simulink model "SSBWeaverModulatorandDemodulator"  (R2021a)
settings: Solver=VariableStepAuto  StartTime=0.0  StopTime=1  RelTol=1e-3
libraries: dspfdesign x4
settings Model: Creator=ZephyrY  LastModifiedBy=ZephyrY

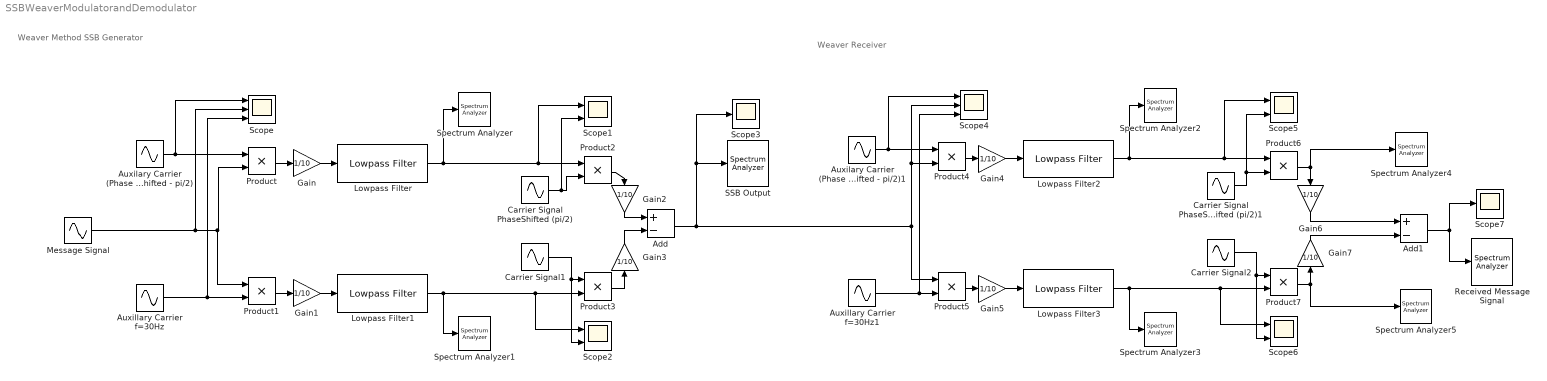
== system SSBWeaverModulatorandDemodulator ==
  note: Weaver Receiver
  note: Weaver Method
      | SSB Generator
  Add : Sum  Inputs=+-
  Add1 : Sum  Inputs=+-
  Auxilary Carrier (Phase Shifted - pi/2) : Sin  Amplitude=10  Frequency=2*pi*30  Phase=pi  SampleTime=1e-3
  Auxilary Carrier (Phase Shifted - pi/2)1 : Sin  Amplitude=10  Frequency=2*pi*30  Phase=pi  SampleTime=1e-3
  Auxillary Carrier f=30Hz : Sin  Amplitude=10  Frequency=2*pi*30  Phase=pi/2  SampleTime=1e-3
  Auxillary Carrier f=30Hz1 : Sin  Amplitude=10  Frequency=2*pi*30  Phase=pi/2  SampleTime=1e-3
  Carrier Signal PhaseShifted (pi/2) : Sin  Amplitude=10  Frequency=2*pi*100  Phase=pi  SampleTime=1e-3
  Carrier Signal PhaseShifted (pi/2)1 : Sin  Amplitude=10  Frequency=2*pi*100  Phase=pi  SampleTime=1e-3
  Carrier Signal1 : Sin  Amplitude=10  Frequency=2*pi*100  Phase=pi/2  SampleTime=1e-3
  Carrier Signal2 : Sin  Amplitude=10  Frequency=2*pi*100  Phase=pi/2  SampleTime=1e-3
  Gain{,1..7} (8 alike) : Gain  Gain=1/10
  Lowpass Filter : dspfdesign/Lowpass Filter  FilterType=FIR  DesignForMinimumOrder=off  FilterOrder=200  PassbandFrequency=25  StopbandFrequency=12e3  PassbandRipple=0.1  StopbandAttenuation=80  InheritSampleRate=on  SampleRate=44100  SimulateUsing=Interpreted execution  roundingMode=Floor  coeffsDataTypeStr=fixdt(1,16)
  Lowpass Filter1 : dspfdesign/Lowpass Filter  FilterType=FIR  DesignForMinimumOrder=off  FilterOrder=200  PassbandFrequency=25  StopbandFrequency=12e3  PassbandRipple=0.1  StopbandAttenuation=80  InheritSampleRate=on  SampleRate=44100  SimulateUsing=Interpreted execution  roundingMode=Floor  coeffsDataTypeStr=fixdt(1,16)
  Lowpass Filter2 : dspfdesign/Lowpass Filter  FilterType=FIR  DesignForMinimumOrder=off  FilterOrder=200  PassbandFrequency=95  StopbandFrequency=12e3  PassbandRipple=0.1  StopbandAttenuation=80  InheritSampleRate=on  SampleRate=44100  SimulateUsing=Interpreted execution  roundingMode=Floor  coeffsDataTypeStr=fixdt(1,16)
  Lowpass Filter3 : dspfdesign/Lowpass Filter  FilterType=FIR  DesignForMinimumOrder=off  FilterOrder=200  PassbandFrequency=95  StopbandFrequency=12e3  PassbandRipple=0.1  StopbandAttenuation=80  InheritSampleRate=on  SampleRate=44100  SimulateUsing=Interpreted execution  roundingMode=Floor  coeffsDataTypeStr=fixdt(1,16)
  Message Signal : Sin  Amplitude=5  Frequency=2*pi*10  Phase=pi/2  SampleTime=1e-3
  Product{,1..7} (8 alike) : Product
  Received Message Signal : SpectrumAnalyzer
  SSB Output : SpectrumAnalyzer
  Scope : Scope  NumInputPorts=3
  Scope{1..2,5..6} (4 alike) : Scope  NumInputPorts=2
  Scope3 : Scope
  Scope4 : Scope  NumInputPorts=3
  Scope7 : Scope
  Spectrum Analyzer{,1..5} (6 alike) : SpectrumAnalyzer
  wires:
  Auxilary Carrier (Phase Shifted - pi/2)/1 -> Scope/1, Product/1
  Message Signal/1 -> Scope/2, Product1/1, Product/2
  Auxillary Carrier f=30Hz/1 -> Scope/3, Product1/2
  Product/1 -> Gain/1
  Product1/1 -> Gain1/1
  Lowpass Filter/1 -> Scope1/1, Product2/1, Spectrum Analyzer/1
  Lowpass Filter1/1 -> Spectrum Analyzer1/1, Scope2/1, Product3/2
  Carrier Signal PhaseShifted (pi/2)/1 -> Scope1/2, Product2/2
  Carrier Signal1/1 -> Scope2/2, Product3/1
  Product2/1 -> Gain2/1
  Product3/1 -> Gain3/1
  Add1/1 -> Scope7/1, Received Message Signal/1
  Lowpass Filter2/1 -> Scope5/1, Product6/1, Spectrum Analyzer2/1
  Auxilary Carrier (Phase Shifted - pi/2)1/1 -> Scope4/1, Product4/1
  Carrier Signal PhaseShifted (pi/2)1/1 -> Scope5/2, Product6/2
  Add/1 -> Product5/1, Scope4/2, Product4/2, Scope3/1, SSB Output/1
  Auxillary Carrier f=30Hz1/1 -> Scope4/3, Product5/2
  Product7/1 -> Spectrum Analyzer5/1, Gain7/1
  Lowpass Filter3/1 -> Spectrum Analyzer3/1, Scope6/1, Product7/2
  Carrier Signal2/1 -> Scope6/2, Product7/1
  Product6/1 -> Gain6/1, Spectrum Analyzer4/1
  Gain/1 -> Lowpass Filter/1
  Gain1/1 -> Lowpass Filter1/1
  Gain2/1 -> Add/1
  Gain3/1 -> Add/2
  Product4/1 -> Gain4/1
  Gain4/1 -> Lowpass Filter2/1
  Product5/1 -> Gain5/1
  Gain5/1 -> Lowpass Filter3/1
  Gain6/1 -> Add1/1
  Gain7/1 -> Add1/2
